simulink model "sim_quadrotor_2018"  (R2018a)
settings: Solver=ode3  StartTime=0  StopTime=inf  FixedStep=quadEDT.sampletime  MaxStep=0.1  RelTol=1e-3  EnableMultiTasking=on
InitFcn:
  | % load parameters of the default quadrotor
  | disp('Quadrotor parameters loaded by InitFcn')
  | parameters_estimationcontrol %loads mdl_quadcopter, too!
  | 
  | % change to Simulation folder if in data folder
  | %cd([matlabpath '/Simulation']);
  | cd(['C:\Users\Tony\Documents\GitHub\drone\MIT_MatlabToolbox\trunk\matlab\Simulation']);
StopFcn:
  | SimulationDataToHardwareDataFormat
values from neighbouring files (symbols this model uses):
  controlHelperParams =     [LQR_param.mat]
  dT = quadEDT.sampletime    [parameters_estimationcontrol.m]
  estimParams =     [LQR_param.mat]
  quad =     [LQR_param.mat]
  quadEDT =     [LQR_param.mat]
  sigmaW = blkdiag(0.0005, 0.1)    [parameters_estimationcontrol.m]
  sigmaX0 = zeros(2,2)    [parameters_estimationcontrol.m]
  x0 = [-0.05 0]    [parameters_estimationcontrol.m]
undefined symbols (not defined in the file or in its folder): DiscIntNeverNeededParam, Discrete, Time
libraries: simulink x28, dspswit3 x6, ctrlSharedLib x3, vrlib x1, commnoisgen2 x1
(part 1 of 2)
settings Model: Creator=Fabian Riether  LastModifiedBy=Tony
settings SolverCC: ConcurrentTasks=on  AutoInsertRateTranBlk=on
settings DataIOCC: SaveFormat=StructureWithTime  SignalLoggingSaveFormat=ModelDataLogs  SignalLogging=off  DSMLogging=off
settings OptimizationCC: ExpressionDepthLimit=2147483647  LifeSpan=1
settings DebuggingCC: UnderspecifiedInitializationDetection=Classic  MergeDetectMultiDrivingBlocksExec=none  SolverPrmCheckMsg=warning  FcnCallInpInsideContextMsg=warning  StateNameClashWarn=warning  SFUnexpectedBacktrackingDiag=warning  SFNoUnconditionalDefaultTransitionDiag=warning  SFExecutionAtInitializationDiag=none
settings HardwareCC: ProdBitPerPointer=32  ProdBitPerSizeT=32  ProdBitPerPtrDiffT=32  ProdLargestAtomicFloat=None  ProdIntDivRoundTo=Undefined  ProdEndianess=Unspecified  ProdWordSize=32  ProdHWDeviceType=32-bit Generic  TargetBitPerPointer=64  TargetBitPerSizeT=64  TargetBitPerPtrDiffT=64  TargetLongLongMode=on  TargetIntDivRoundTo=Zero  TargetEndianess=LittleEndian  TargetWordSize=64  TargetHWDeviceType=MATLAB Host  ProdEqTarget=off
settings ModelReferenceCC: PropagateSignalLabelsOutOfModel=off
settings SFSimCC: MATLABDynamicMemAlloc=off
settings RTWCC: SystemTargetFile=ert_shrlib.tlc  GenCodeOnly=on  MakeCommand="make_rtw OPTS=\"-DDEFAULT_BUFFER_SIZE=4600\""  GenerateMakefile=off  TemplateMakefile=ert_default_tmf  Description=Embedded Coder (host-based shared library target)  BuildConfiguration=Faster Runs  RTWCompilerOptimization=on
settings CodeAppCC: IgnoreCustomStorageClasses=off  StateflowObjectComments=on
settings STFCustomTargetCC: GenerateSampleERTMain=on  ParMdlRefBuildCompliant=on  CompOptLevelCompliant=on  IncludeMdlTerminateFcn=off  CombineOutputUpdateFcns=on  ERTCustomFileBanners=on  MatFileLogging=on  MultiInstanceERTCode=on  CodeInterfacePackaging=Reusable function  SupportContinuousTime=off  SupportNonInlinedSFcns=off  RemoveResetFunc=on  MATLABClassNameForMDSCustomization=Simulink.SoftwareTarget.ERTCustomization  ModelStepFunctionPrototypeControlCompliant=on  GRTInterface=off  UseToolchainInfoCompliant=on  SystemTargetFile=ert_shrlib.tlc
settings ERTTargetCC: MultiwordLength=2048  GenerateSampleERTMain=on  ConcurrentExecutionCompliant=off  IncludeMdlTerminateFcn=off  MatFileLogging=on  MultiInstanceERTCode=on  CodeInterfacePackaging=Reusable function  CPPClassGenCompliant=off  MultiInstanceErrorCode=Warning  ERTCustomFileTemplate=example_file_process.tlc  ConvertIfToSwitch=off  SuppressUnreachableDefaultCases=off
settings ConfigComp: CovMetricSettings=dw  CovHtmlReporting=on  CovSaveCumulativeToWorkspaceVar=on  CovSaveSingleToWorkspaceVar=on  CovExternalEMLEnable=off  CovSFcnEnable=off

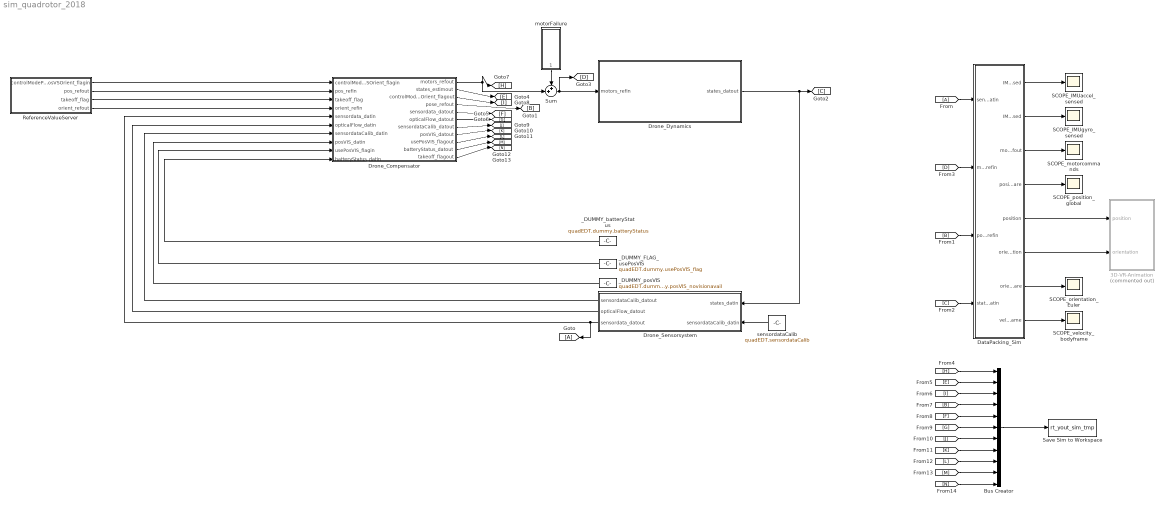
== system sim_quadrotor_2018 ==
  3D-VR-Animation : Subsystem  Commented=on
  Bus Creator : BusCreator  Inputs=11
  DataPacking_Sim : Subsystem
  Drone_Compensator : Subsystem  TreatAsAtomicUnit=on
  Drone_Dynamics : Subsystem  AncestorBlock=roblocks/Dynamics/Quadrotor
  Drone_Sensorsystem : Subsystem
  ReferenceValueServer : Subsystem
  SCOPE_IMUaccel_sensed : Scope
  SCOPE_IMUgyro_sensed : Scope
  SCOPE_motorcommands : Scope
  SCOPE_orientation_Euler : Scope
  SCOPE_position_global : Scope
  SCOPE_velocity_bodyframe : Scope
  Save Sim to Workspace : ToWorkspace  VariableName=rt_yout_sim_tmp  SaveFormat=Timeseries  SampleTime=-1
  Sum : Sum  Inputs=++|
  _DUMMY_FLAG_usePosVIS : Constant  Value=quadEDT.dummy.usePosVIS_flag
  _DUMMY_batteryStatus : Constant  Value=quadEDT.dummy.batteryStatus
  _DUMMY_posVIS : Constant  Value=quadEDT.dummy.posVIS_novisionavail
  motorFailure : Subsystem
  sensordataCalib : Constant  Value=quadEDT.sensordataCalib  SampleTime=quadEDT.sampletime
  wires:
  ReferenceValueServer/2("pos_refout ") -> Drone_Compensator/2(pos_refin)
  Sum/1 -> [D], Drone_Dynamics/1(motors_refin)
  motorFailure/1(motors_datout) -> Sum/1
  Drone_Compensator/1(motors_refout) -> [H], Sum/2
  ReferenceValueServer/1(controlModePosVSOrient_flagin) -> Drone_Compensator/1(controlModePosVSOrient_flagin)
  ReferenceValueServer/4(orient_refout) -> Drone_Compensator/4(orient_refin)
  Drone_Dynamics/1(states_datout) -> [C], Drone_Sensorsystem/1(states_datin)
  sensordataCalib/1 -> Drone_Sensorsystem/2(sensordataCalib_datin)
  Drone_Sensorsystem/2(opticalFlow_datout) -> Drone_Compensator/6(opticalFlow_datin)
  Drone_Sensorsystem/1(sensordataCalib_datout) -> Drone_Compensator/7(sensordataCalib_datin)
  Drone_Sensorsystem/3(sensordata_datout) -> [A], Drone_Compensator/5(sensordata_datin)
  _DUMMY_posVIS/1 -> Drone_Compensator/8(posVIS_datin)
  _DUMMY_FLAG_usePosVIS/1 -> Drone_Compensator/9(usePosVIS_flagin)
  _DUMMY_batteryStatus/1 -> Drone_Compensator/10(batteryStatus_datin)
  ReferenceValueServer/3("takeoff_flag ") -> Drone_Compensator/3(takeoff_flag)
  Drone_Compensator/4(pose_refout) -> [B]
  [A] -> DataPacking_Sim/1(sensordata_datin)
  [B] -> DataPacking_Sim/3(pose_refin)
  [C] -> DataPacking_Sim/4(states_datin)
  DataPacking_Sim/1(IMUaccel_sensed) -> SCOPE_IMUaccel_sensed/1
  DataPacking_Sim/2(IMUgyro_sensed) -> SCOPE_IMUgyro_sensed/1
  DataPacking_Sim/4(position_compare) -> SCOPE_position_global/1
  DataPacking_Sim/5(position) -> 3D-VR-Animation/1(position)
  DataPacking_Sim/7(orientation_compare) -> SCOPE_orientation_Euler/1
  DataPacking_Sim/6(orientation) -> 3D-VR-Animation/2(orientation)
  [D] -> DataPacking_Sim/2(motors_refin)
  DataPacking_Sim/3(motors_refout) -> SCOPE_motorcommands/1
  DataPacking_Sim/8(velocity_bodyframe) -> SCOPE_velocity_bodyframe/1
  Drone_Compensator/2(states_estimout) -> [E]
  Drone_Compensator/5(sensordata_datout) -> [F]
  Drone_Compensator/6(opticalFlow_datout) -> [G]
  Drone_Compensator/7(sensordataCalib_datout) -> [J]
  Drone_Compensator/8(posVIS_datout) -> [K]
  Drone_Compensator/9(usePosVIS_flagout) -> [L]
  Drone_Compensator/10(batteryStatus_datout) -> [M]
  [H] -> Bus Creator/1
  [E] -> Bus Creator/2
  [I] -> Bus Creator/3
  [B] -> Bus Creator/4
  [F] -> Bus Creator/5
  [G] -> Bus Creator/6
  [J] -> Bus Creator/7
  [K] -> Bus Creator/8
  [L] -> Bus Creator/9
  [M] -> Bus Creator/10
  [N] -> Bus Creator/11
  Bus Creator/1 -> Save Sim to Workspace/1
  Drone_Compensator/3(controlModePosVSOrient_flagout) -> [I]
  Drone_Compensator/11(takeoff_flagout) -> [N]

== system sim_quadrotor_2018/3D-VR-Animation ==
  note: Student contribution by Erlend Solbakk Harbitz
  note: In animation:
      | X-axis: red
      | Y-axis: green
      | Z-axis: blue
  note: Animation
  note: Positions = [X; Y; Z] (Inertia frame with Z-axis downwards)
      | Theta      = [yaw (psi); pitch ( theta); roll (phi) ]
      |
      | Euler angles scheme: First yaw, then pitch, then roll
  position : Inport
  orientation : Inport  Port=2
  Double click for animation : vrlib/VR Sink  RequirementInfo={} %GIDa_850cb678_ba1c_4e80_94b9_fad132a707ef  InstantiateOnLoad=on  SampleTime=0.1  ViewEnable=on  RemoteChange=off  RemoteView=off  FieldsWritten=DRONE.translation.3.1.1.double#roll_rotation.rotation.4.1.1.double#pitch_rotation.rotation.4.1.1.double#yaw_rotation.rotation.4.1.1.double  WorldFileName=Animation/DroneWorld.wrl  AutoView=off  VideoDimensions=[]  AllowVariableSize=off
      settings: SourceProductBaseCode=VR
  Euler angle rotations : MATLAB Function  TreatAsAtomicUnit=on
  Rate Transition : RateTransition
  Rate Transition1 : RateTransition
  wires:
  orientation/1 -> Rate Transition1/1  "Euler angles (yaw, pitch, roll)"
  position/1 -> Rate Transition/1  "Inertia positions X,Y,Z"
  Rate Transition1/1 -> Euler angle rotations/1(O)
  Rate Transition/1 -> Double click for animation/1
  Euler angle rotations/1(rot_phi) -> Double click for animation/2  "Third rotation"
  Euler angle rotations/2(rot_theta) -> Double click for animation/3  "Second rotation"
  Euler angle rotations/3(rot_psi) -> Double click for animation/4  "First rotation"

== system sim_quadrotor_2018/DataPacking_Sim ==
  sensordata_datin : Inport
  motors_refin : Inport  Port=2
  pose_refin : Inport  Port=3
  states_datin : Inport  Port=4
  Augment/Mux Signals : Subsystem
  Bus Selector1 : BusSelector  OutputSignals=dx,dy,dz  OutputAsBus=on
  Bus Selector6 : BusSelector  OutputSignals=ddx,ddy,ddz  OutputAsBus=on
  Bus Selector9 : BusSelector  OutputSignals=p,q,r  OutputAsBus=on
  IMUaccel_sensed : Outport
  IMUgyro_sensed : Outport  Port=2
  motors_refout : Outport  Port=3
  position_compare : Outport  Port=4
  position : Outport  Port=5
  orientation : Outport  Port=6
  orientation_compare : Outport  Port=7
  velocity_bodyframe : Outport  Port=8
  wires:
  sensordata_datin/1 -> Bus Selector6/1, Bus Selector9/1
  states_datin/1 -> Bus Selector1/1, Augment/Mux Signals/2(states_datin)
  pose_refin/1 -> Augment/Mux Signals/1(pose_refin)
  Bus Selector9/1 -> IMUgyro_sensed/1
  Bus Selector6/1 -> IMUaccel_sensed/1
  Augment/Mux Signals/1(position_compare_datout) -> position_compare/1
  Augment/Mux Signals/2(position_datout) -> position/1
  Augment/Mux Signals/3(orientation_compare_datout) -> orientation_compare/1
  Augment/Mux Signals/4(orientation_datout) -> orientation/1
  motors_refin/1 -> motors_refout/1
  Bus Selector1/1 -> velocity_bodyframe/1

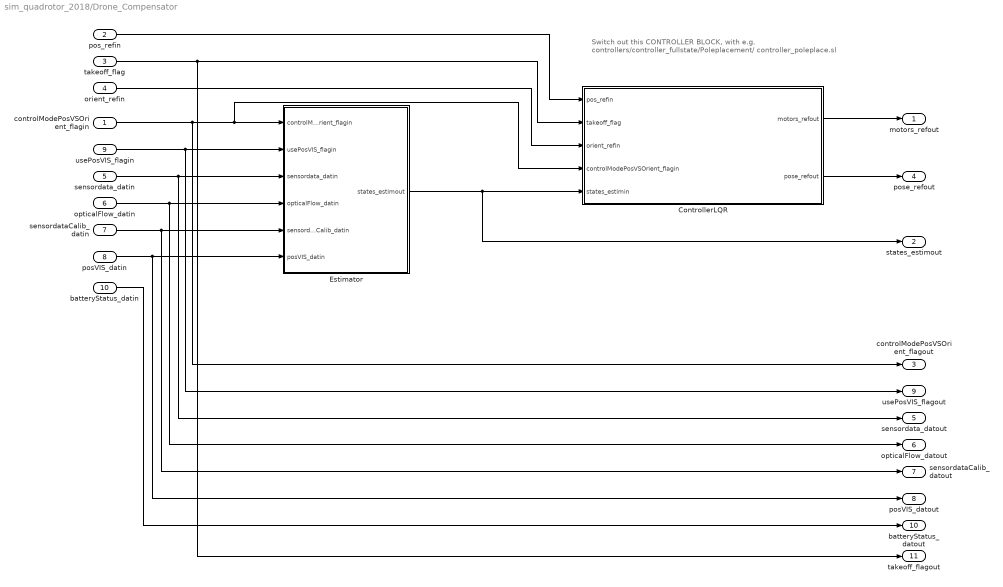
== system sim_quadrotor_2018/Drone_Compensator ==
  note: Switch out this CONTROLLER BLOCK, with e.g.
      | controllers/controller_fullstate/Poleplacement/
      | controller_poleplace.sl
  controlModePosVSOrient_flagin : Inport
  pos_refin : Inport  Port=2
  takeoff_flag : Inport  Port=3
  orient_refin : Inport  Port=4
  sensordata_datin : Inport  Port=5
  opticalFlow_datin : Inport  Port=6
  sensordataCalib_datin : Inport  Port=7
  posVIS_datin : Inport  Port=8
  usePosVIS_flagin : Inport  Port=9
  batteryStatus_datin : Inport  Port=10
  ControllerLQR : Subsystem  TreatAsAtomicUnit=on
  Estimator : Subsystem
  motors_refout : Outport
  states_estimout : Outport  Port=2
  controlModePosVSOrient_flagout : Outport  Port=3
  pose_refout : Outport  Port=4
  sensordata_datout : Outport  Port=5
  opticalFlow_datout : Outport  Port=6
  sensordataCalib_datout : Outport  Port=7
  posVIS_datout : Outport  Port=8
  usePosVIS_flagout : Outport  Port=9
  batteryStatus_datout : Outport  Port=10
  takeoff_flagout : Outport  Port=11
  wires:
  sensordata_datin/1 -> sensordata_datout/1, Estimator/3(sensordata_datin)
  pos_refin/1 -> ControllerLQR/1(pos_refin)
  Estimator/1(states_estimout) -> ControllerLQR/5(states_estimin), states_estimout/1
  orient_refin/1 -> ControllerLQR/3(orient_refin)
  controlModePosVSOrient_flagin/1 -> controlModePosVSOrient_flagout/1, ControllerLQR/4(controlModePosVSOrient_flagin), Estimator/1(controlModePosVSOrient_flagin)
  sensordataCalib_datin/1 -> sensordataCalib_datout/1, Estimator/5(sensordataCalib_datin)
  opticalFlow_datin/1 -> opticalFlow_datout/1, Estimator/4(opticalFlow_datin)
  posVIS_datin/1 -> posVIS_datout/1, Estimator/6(posVIS_datin)
  ControllerLQR/1(motors_refout) -> motors_refout/1
  usePosVIS_flagin/1 -> usePosVIS_flagout/1, Estimator/2(usePosVIS_flagin)
  ControllerLQR/2(pose_refout) -> pose_refout/1
  batteryStatus_datin/1 -> batteryStatus_datout/1
  takeoff_flag/1 -> ControllerLQR/2(takeoff_flag), takeoff_flagout/1

== system sim_quadrotor_2018/Drone_Dynamics ==
  motors_refin : Inport
  Bus Creator : BusCreator  Inputs='X','Y','Z','yaw','pitch','roll','dx','dy','dz','p','q','r'
  Demux : Demux  Outputs=12
  Dynamics (Robotics Toolbox Peter Corke) : S-Function  FunctionName=quadrotor_dynamics  Parameters=quad  SFunctionDeploymentMode=off  EnableBusSupport=off
  MotorsToW : Subsystem
  Rate Transition : RateTransition
  states_datout : Outport
  wires:
  Demux/1 -> Bus Creator/1  "X"
  Demux/3 -> Bus Creator/3  "Z"
  Demux/4 -> Bus Creator/4  "yaw"
  Demux/5 -> Bus Creator/5  "pitch"
  motors_refin/1 -> Rate Transition/1
  Demux/7 -> Bus Creator/7  "dx"
  Demux/9 -> Bus Creator/9  "dz"
  Demux/2 -> Bus Creator/2  "Y"
  Demux/6 -> Bus Creator/6  "roll"
  Demux/8 -> Bus Creator/8  "dy"
  Bus Creator/1 -> states_datout/1
  Dynamics (Robotics Toolbox Peter Corke)/1 -> Demux/1
  Demux/10 -> Bus Creator/10  "p"
  Demux/11 -> Bus Creator/11  "q"
  Demux/12 -> Bus Creator/12  "r"
  MotorsToW/1(omegas_datout) -> Dynamics (Robotics Toolbox Peter Corke)/1
  Rate Transition/1 -> MotorsToW/1(motors_datin)

== system sim_quadrotor_2018/Drone_Sensorsystem ==
  states_datin : Inport
  sensordataCalib_datin : Inport  Port=2
  IMU_Pressure : Subsystem
  Rate Transition1 : RateTransition  OutPortSampleTime=quadEDT.sampletime
  Rate Transition2 : RateTransition  OutPortSampleTime=quadEDT.sampletime
  camera : Subsystem
  sensordataCalib_datout : Outport
  opticalFlow_datout : Outport  Port=2
  sensordata_datout : Outport  Port=3
  wires:
  states_datin/1 -> IMU_Pressure/2(states_datin), camera/1(states_datin)
  sensordataCalib_datin/1 -> sensordataCalib_datout/1, IMU_Pressure/1(sensordataCalib_datin)
  Rate Transition2/1 -> sensordata_datout/1
  Rate Transition1/1 -> opticalFlow_datout/1
  IMU_Pressure/1(sensordata_datout) -> Rate Transition2/1
  camera/1(opticalFlow_datout) -> Rate Transition1/1

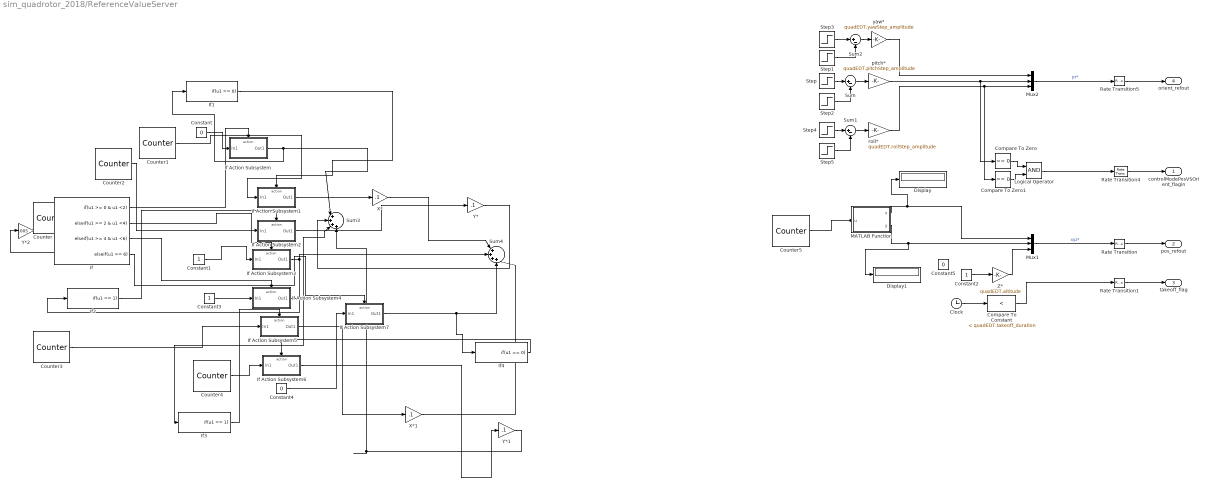
== system sim_quadrotor_2018/ReferenceValueServer ==
  Clock : Clock
  Compare To Constant : simulink/Logic and Bit Operations/Compare To Constant  relop=<  const=quadEDT.takeoff_duration  OutDataTypeStr=boolean
  Compare To Zero : simulink/Logic and Bit Operations/Compare To Zero  relop===  OutDataTypeStr=boolean
  Compare To Zero1 : simulink/Logic and Bit Operations/Compare To Zero  relop===  OutDataTypeStr=boolean
  Constant : Constant  Value=0  SampleTime=0
  Constant1 : Constant  SampleTime=0
  Constant2 : Constant  SampleTime=0
  Constant3 : Constant  SampleTime=0
  Constant4 : Constant  Value=0  SampleTime=0
  Constant5 : Constant  Value=0  SampleTime=0
  Counter : dspswit3/Counter  Direction=Up  CountEvent=Free running  CounterSize=User defined  MaxCount=1600  InitialCount=0  Output=Count  HitValue=32  ResetInput=on  SamplesPerFrame=1  Ts=.005  CntDtype=double  HitDtype=Logical
  Counter1 : dspswit3/Counter  Direction=Up  CountEvent=Free running  CounterSize=User defined  MaxCount=10  InitialCount=0  Output=Count  HitValue=32  ResetInput=on  SamplesPerFrame=1  Ts=.005  CntDtype=double  HitDtype=Logical
  Counter2 : dspswit3/Counter  Direction=Up  CountEvent=Free running  CounterSize=User defined  MaxCount=10  InitialCount=0  Output=Count  HitValue=32  ResetInput=on  SamplesPerFrame=1  Ts=.005  CntDtype=double  HitDtype=Logical
  Counter3 : dspswit3/Counter  Direction=Down  CountEvent=Free running  CounterSize=User defined  MaxCount=10  InitialCount=10  Output=Count  HitValue=32  ResetInput=on  SamplesPerFrame=1  Ts=.005  CntDtype=double  HitDtype=Logical
  Counter4 : dspswit3/Counter  Direction=Down  CountEvent=Free running  CounterSize=User defined  MaxCount=10  InitialCount=10  Output=Count  HitValue=32  ResetInput=on  SamplesPerFrame=1  Ts=.005  CntDtype=double  HitDtype=Logical
  Counter5 : dspswit3/Counter  Direction=Up  CountEvent=Free running  CounterSize=User defined  MaxCount=10000000000000000000000000000000000000000  InitialCount=0  Output=Count  HitValue=32  ResetInput=off  SamplesPerFrame=1  Ts=.005  CntDtype=double  HitDtype=Logical
  Display : Display
      settings: Decimation=2
  Display1 : Display
      settings: Decimation=2
  If : If  IfExpression=u1 >= 0 & u1 <2  ElseIfExpressions=u1 >= 2 & u1 <4,u1 >= 4 & u1 <6,u1 >= 6  ShowElse=off
  If Action Subsystem : Subsystem  TreatAsAtomicUnit=on
  If Action Subsystem1 : Subsystem  TreatAsAtomicUnit=on
  If Action Subsystem2 : Subsystem  TreatAsAtomicUnit=on
  If Action Subsystem3 : Subsystem  TreatAsAtomicUnit=on
  If Action Subsystem4 : Subsystem  TreatAsAtomicUnit=on
  If Action Subsystem5 : Subsystem  TreatAsAtomicUnit=on
  If Action Subsystem6 : Subsystem  TreatAsAtomicUnit=on
  If Action Subsystem7 : Subsystem  TreatAsAtomicUnit=on
  If1 : If  IfExpression=u1 == 0  ShowElse=off
  If2 : If  IfExpression=u1 == 1  ShowElse=off
  If3 : If  IfExpression=u1 == 1  ShowElse=off
  If4 : If  IfExpression=u1 == 0  ShowElse=off
  Logical Operator : Logic  AllPortsSameDT=off  OutDataTypeStr=boolean
  MATLAB Function : MATLAB Function  TreatAsAtomicUnit=on
  Mux1 : Mux  Inputs=3
  Mux2 : Mux  Inputs=3
  Rate Transition{,1,4..5} (4 alike) : RateTransition  OutPortSampleTime=quadEDT.sampletime
  Step : Step  Time=quadEDT.pitchStep_time  SampleTime=0
  Step1 : Step  Time=quadEDT.yawStep_time+quadEDT.yawStep_duration  SampleTime=0
  Step2 : Step  Time=quadEDT.pitchStep_time+quadEDT.pitchStep_duration  SampleTime=0
  Step3 : Step  Time=quadEDT.yawStep_time  SampleTime=0
  Step4 : Step  Time=quadEDT.rollStep_time  SampleTime=0
  Step5 : Step  Time=quadEDT.rollStep_duration+quadEDT.rollStep_time  SampleTime=0
  Sum : Sum  Inputs=|+-
  Sum1 : Sum  Inputs=|+-
  Sum2 : Sum  Inputs=|+-
  Sum3 : Sum  Inputs=|++++
  Sum4 : Sum  Inputs=|++++
  X* : Gain  Gain=.1
  X*1 : Gain  Gain=.1
  Y* : Gain  Gain=.1
  Y*1 : Gain  Gain=.1
  Y*2 : Gain  Gain=.005
  Z* : Gain  Gain=quadEDT.altitude
  pitch* : Gain  Gain=quadEDT.pitchStep_amplitude
  roll* : Gain  Gain=quadEDT.rollStep_amplitude
  yaw* : Gain  Gain=quadEDT.yawStep_amplitude
  controlModePosVSOrient_flagin : Outport
  "pos_refout " : Outport  Port=2
  "takeoff_flag " : Outport  Port=3
  orient_refout : Outport  Port=4
  wires:
  Constant/1 -> If Action Subsystem/1(In1)
  Mux1/1 -> Rate Transition/1  "xyz*"
  Rate Transition/1 -> "pos_refout "/1
  Rate Transition4/1 -> controlModePosVSOrient_flagin/1
  Step/1 -> Sum/1
  Mux2/1 -> Rate Transition5/1  "pr*"
  Sum1/1 -> roll*/1
  Rate Transition5/1 -> orient_refout/1
  Sum/1 -> pitch*/1
  Step2/1 -> Sum/2
  yaw*/1 -> Mux2/1
  pitch*/1 -> Mux2/2, Compare To Zero/1
  roll*/1 -> Mux2/3, Compare To Zero1/1
  Compare To Zero/1 -> Logical Operator/1
  Compare To Zero1/1 -> Logical Operator/2
  Logical Operator/1 -> Rate Transition4/1
  Clock/1 -> Compare To Constant/1
  Constant2/1 -> Z*/1
  Z*/1 -> Mux1/3
  Step4/1 -> Sum1/1
  Step5/1 -> Sum1/2
  Sum2/1 -> yaw*/1
  Step3/1 -> Sum2/1
  Step1/1 -> Sum2/2
  Compare To Constant/1 -> Rate Transition1/1
  Rate Transition1/1 -> "takeoff_flag "/1
  Constant1/1 -> If Action Subsystem3/1(In1)
  If Action Subsystem/1(Out1) -> If1/1, Sum3/1
  If Action Subsystem1/1(Out1) -> X*/1
  Counter/1 -> Y*2/1
  Counter1/1 -> If Action Subsystem1/1(In1)
  If/1 -> If Action Subsystem/Action
  Counter2/1 -> If Action Subsystem2/1(In1)
  If/2 -> If Action Subsystem3/Action
  If Action Subsystem3/1(Out1) -> If2/1, Sum4/2
  If Action Subsystem2/1(Out1) -> Y*/1
  If/3 -> If Action Subsystem4/Action
  Constant3/1 -> If Action Subsystem4/1(In1)
  Counter3/1 -> If Action Subsystem5/1(In1)
  If Action Subsystem4/1(Out1) -> If3/1, Sum3/3
  If Action Subsystem5/1(Out1) -> X*1/1
  If/4 -> If Action Subsystem7/Action
  Counter4/1 -> If Action Subsystem6/1(In1)
  If Action Subsystem6/1(Out1) -> Y*1/1
  If Action Subsystem7/1(Out1) -> If4/1, Sum4/4
  Constant4/1 -> If Action Subsystem7/1(In1)
  If1/1 -> If Action Subsystem1/Action
  If2/1 -> If Action Subsystem2/Action
  If3/1 -> If Action Subsystem5/Action
  If4/1 -> If Action Subsystem6/Action
  X*/1 -> Sum4/1
  X*1/1 -> Sum4/3
  Y*/1 -> Sum3/2
  Y*1/1 -> Sum3/4
  Y*2/1 -> If/1
  Counter5/1 -> MATLAB Function/1(u)
  MATLAB Function/2(y) -> Display1/1, Mux1/2
  MATLAB Function/1(x) -> Display/1, Mux1/1

== system sim_quadrotor_2018/motorFailure ==
  Mux1 : Mux
  Step : Step  Time=quadEDT.motorFailure_time  SampleTime=quadEDT.sampletime
  Step1 : Step  Time=quadEDT.motorFailure_time + quadEDT.motorFailure_duration  SampleTime=quadEDT.sampletime
  Sum : Sum  Inputs=|+-
  motorFailure_gainm1 : Gain  Gain=quadEDT.motorFailure_m2
  motorFailure_gainm2 : Gain  Gain=quadEDT.motorFailure_m2
  motorFailure_gainm3 : Gain  Gain=quadEDT.motorFailure_m3
  motorFailure_gainm4 : Gain  Gain=quadEDT.motorFailure_m3
  motors_datout : Outport
  wires:
  Step/1 -> Sum/1
  Step1/1 -> Sum/2
  Sum/1 -> motorFailure_gainm1/1, motorFailure_gainm2/1, motorFailure_gainm3/1, motorFailure_gainm4/1
  motorFailure_gainm2/1 -> Mux1/2
  motorFailure_gainm3/1 -> Mux1/3
  motorFailure_gainm4/1 -> Mux1/4
  motorFailure_gainm1/1 -> Mux1/1
  Mux1/1 -> motors_datout/1

== system sim_quadrotor_2018/DataPacking_Sim/Augment//Mux Signals ==
  pose_refin : Inport
  states_datin : Inport  Port=2
  Bus Selector7 : BusSelector  OutputSignals=X,Y,Z  OutputAsBus=on
  Bus Selector8 : BusSelector  OutputSignals=yaw,pitch,roll  OutputAsBus=on
  Mux : Mux  Inputs=2
  Mux1 : Mux  Inputs=2
  Rate Transition : RateTransition
  orientation_ref : Selector  InputPortWidth=6  IndexOptions=Index vector (dialog)  Indices=[4:6]  OutputSizes=1
  position_ref : Selector  InputPortWidth=6  IndexOptions=Index vector (dialog)  Indices=[1:3]  OutputSizes=1
  position_compare_datout : Outport
  position_datout : Outport  Port=2
  orientation_compare_datout : Outport  Port=3
  orientation_datout : Outport  Port=4
  wires:
  states_datin/1 -> Bus Selector7/1, Bus Selector8/1
  Rate Transition/1 -> orientation_ref/1, position_ref/1
  pose_refin/1 -> Rate Transition/1
  Bus Selector8/1 -> orientation_datout/1, Mux1/2
  Mux1/1 -> orientation_compare_datout/1
  position_ref/1 -> Mux/1
  Mux/1 -> position_compare_datout/1
  orientation_ref/1 -> Mux1/1
  Bus Selector7/1 -> position_datout/1, Mux/2

== system sim_quadrotor_2018/Drone_Compensator/ControllerLQR ==
  pos_refin : Inport
  takeoff_flag : Inport  Port=2
  orient_refin : Inport  Port=3
  controlModePosVSOrient_flagin : Inport  Port=4
  states_estimin : Inport  Port=5
  Add : Sum  Inputs=-+
  FullstateController : Subsystem
  Select pose : Selector  InputPortWidth=12  IndexOptions=Index vector (dialog)  Indices=[1:6]  OutputSizes=1
  SysteminputConverter : Subsystem
  statesReferences : Subsystem
  motors_refout : Outport
  pose_refout : Outport  Port=2
  wires:
  Select pose/1 -> pose_refout/1
  statesReferences/1(states_refout) -> Add/1, Select pose/1
  controlModePosVSOrient_flagin/1 -> statesReferences/3(controlModePosVSOrient_flagin)
  states_estimin/1 -> statesReferences/4(states_estimin), Add/2
  orient_refin/1 -> statesReferences/2(orient_refin)
  pos_refin/1 -> statesReferences/1(pos_refin)
  Add/1 -> FullstateController/1(state_error_datin)  "state error e"
  FullstateController/1(motors_refout) -> SysteminputConverter/2(motors_refin)
  SysteminputConverter/1(motors_refout) -> motors_refout/1
  takeoff_flag/1 -> SysteminputConverter/1(takeoffphase_flagin)

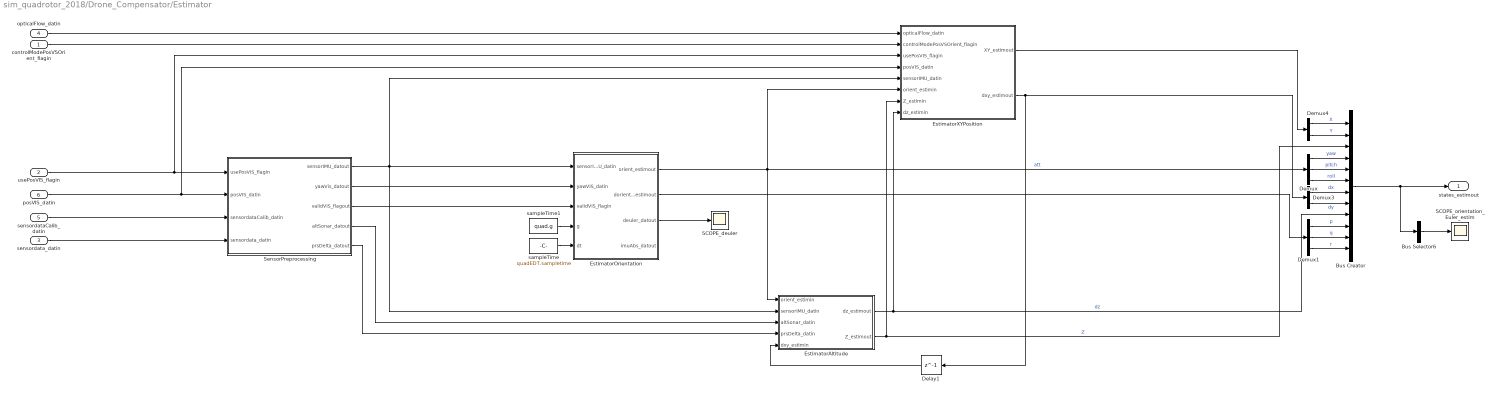
== system sim_quadrotor_2018/Drone_Compensator/Estimator ==
  controlModePosVSOrient_flagin : Inport
  usePosVIS_flagin : Inport  Port=2
  sensordata_datin : Inport  Port=3
  opticalFlow_datin : Inport  Port=4
  sensordataCalib_datin : Inport  Port=5
  posVIS_datin : Inport  Port=6
  Bus Creator : BusCreator  Inputs='X','Y','Z','yaw','pitch','roll','dx','dy','dz','p','q','r'
  Bus Selector6 : BusSelector  OutputSignals=yaw,pitch,roll  OutputAsBus=on
  Delay1 : Delay  DelayLength=1  InitialCondition=0
  Demux : Demux  Outputs=3
  Demux1 : Demux  Outputs=3
  Demux3 : Demux  Outputs=2
  Demux4 : Demux  Outputs=2
  EstimatorAltitude : Subsystem
  EstimatorOrientation : MATLAB Function  TreatAsAtomicUnit=on
  EstimatorXYPosition : Subsystem
  SCOPE_deuler : Scope
  SCOPE_orientation_Euler_estim : Scope
  SensorPreprocessing : Subsystem
  sampleTime : Constant  Value=quadEDT.sampletime  SampleTime=quadEDT.sampletime
  sampleTime1 : Constant  Value=quad.g  SampleTime=quadEDT.sampletime
  states_estimout : Outport
  wires:
  Bus Creator/1 -> Bus Selector6/1, states_estimout/1
  sampleTime/1 -> EstimatorOrientation/5(dt)
  sensordataCalib_datin/1 -> SensorPreprocessing/3(sensordataCalib_datin)
  EstimatorAltitude/2(Z_estimout) -> Bus Creator/3, EstimatorXYPosition/7(Z_estimin)  "Z"
  EstimatorAltitude/1(dz_estimout) -> EstimatorXYPosition/8(dz_estimin), Bus Creator/9  "dz"
  opticalFlow_datin/1 -> EstimatorXYPosition/1(opticalFlow_datin)
  Demux3/1 -> Bus Creator/7  "dx"
  Demux3/2 -> Bus Creator/8  "dy"
  EstimatorXYPosition/2(dxy_estimout) -> Delay1/1, Demux3/1
  Delay1/1 -> EstimatorAltitude/5(dxy_estimin)
  controlModePosVSOrient_flagin/1 -> EstimatorXYPosition/2(controlModePosVSOrient_flagin)
  Demux4/1 -> Bus Creator/1  "X"
  Demux4/2 -> Bus Creator/2  "Y"
  EstimatorXYPosition/1(XY_estimout) -> Demux4/1
  posVIS_datin/1 -> EstimatorXYPosition/4(posVIS_datin), SensorPreprocessing/2(posVIS_datin)
  usePosVIS_flagin/1 -> SensorPreprocessing/1(usePosVIS_flagin), EstimatorXYPosition/3(usePosVIS_flagin)
  Bus Selector6/1 -> SCOPE_orientation_Euler_estim/1
  SensorPreprocessing/1(sensorIMU_datout) -> EstimatorAltitude/2(sensorIMU_datin), EstimatorOrientation/1(sensorIMU_datin), EstimatorXYPosition/5(sensorIMU_datin)
  sensordata_datin/1 -> SensorPreprocessing/4(sensordata_datin)
  SensorPreprocessing/4(altSonar_datout) -> EstimatorAltitude/3(altSonar_datin)
  SensorPreprocessing/5(prsDelta_datout) -> EstimatorAltitude/4(prsDelta_datin)
  EstimatorOrientation/1(orient_estimout) -> EstimatorAltitude/1(orient_estimin), EstimatorXYPosition/6(orient_estimin), Demux/1  "att"
  Demux/2 -> Bus Creator/5  "pitch"
  Demux1/1 -> Bus Creator/10  "p"
  Demux1/2 -> Bus Creator/11  "q"
  Demux1/3 -> Bus Creator/12  "r"
  EstimatorOrientation/2(dorient_estimout) -> Demux1/1
  SensorPreprocessing/3(validVIS_flagout) -> EstimatorOrientation/3(validVIS_flagin)
  SensorPreprocessing/2(yawVis_datout) -> EstimatorOrientation/2(yawVIS_datin)
  Demux/3 -> Bus Creator/6  "roll"
  Demux/1 -> Bus Creator/4  "yaw"
  EstimatorOrientation/3(deuler_datout) -> SCOPE_deuler/1
  sampleTime1/1 -> EstimatorOrientation/4(g)

== system sim_quadrotor_2018/Drone_Dynamics/MotorsToW ==
  motors_datin : Inport
  Gain : Gain  Gain=quadEDT.motorUnknownGain_gain
  Motordirections : Gain  Gain=[1 -1 1 -1]
  Motordirections1 : Gain  Gain=[1 -1 1 -1]
  Saturation5 : Saturate  UpperLimit=quadEDT.motors_max  LowerLimit=10
  Signed Sqrt : Sqrt  Operator=signedSqrt  SaturateOnIntegerOverflow=on
  motorsToW2_Gain : Gain  Gain=quadEDT.motorcommandToW2_gain
  omegas_datout : Outport
  wires:
  motorsToW2_Gain/1 -> Signed Sqrt/1
  Signed Sqrt/1 -> Gain/1
  motors_datin/1 -> Motordirections/1
  Motordirections/1 -> Saturation5/1
  Saturation5/1 -> Motordirections1/1
  Motordirections1/1 -> motorsToW2_Gain/1
  Gain/1 -> omegas_datout/1

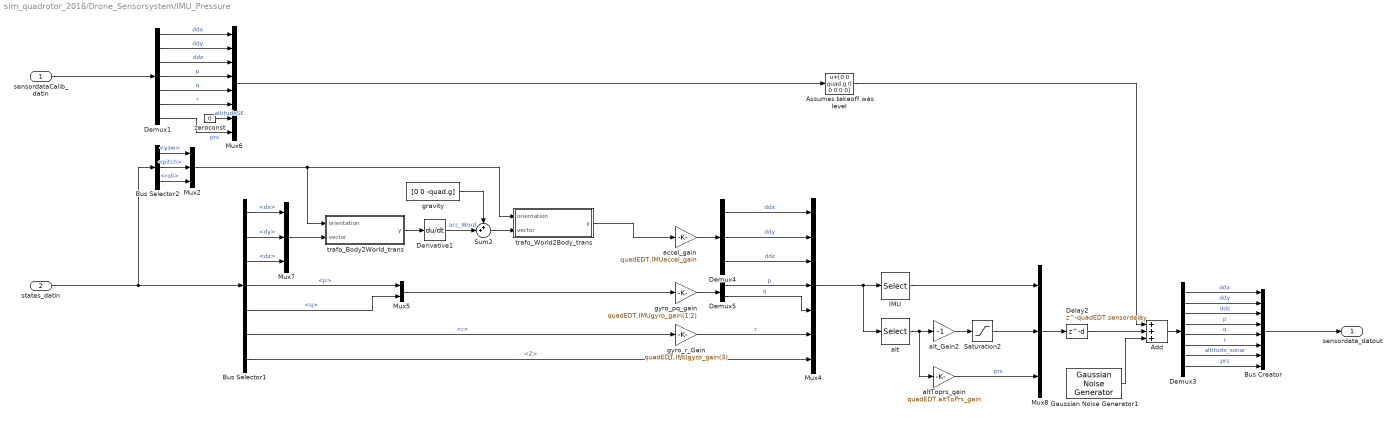
== system sim_quadrotor_2018/Drone_Sensorsystem/IMU_Pressure ==
  sensordataCalib_datin : Inport
  states_datin : Inport  Port=2
  Add : Sum  Inputs=+++
  Assumes takeoff was level : Bias  Bias=[0 0 quad.g 0 0 0 0 0]
  Bus Creator : BusCreator  Inputs=8
  Bus Selector1 : BusSelector  OutputSignals=dx,dy,dz,p,q,r,Z
  Bus Selector2 : BusSelector  OutputSignals=yaw,pitch,roll
  Delay2 : Delay  DelayLength=quadEDT.sensordelay  InitialCondition=0
  Demux1 : Demux  Outputs=7
  Demux3 : Demux  Outputs=8
  Demux4 : Demux  Outputs=3
  Demux5 : Demux  Outputs=2
  Derivative1 : Derivative
  Gaussian Noise Generator1 : commnoisgen2/Gaussian Noise Generator  m=0  d=quadEDT.noiseSensed_var  s=41  Ts=quadEDT.sampletime  frameBased=off  sampPerFrame=1  orient=off  outDataType=double
  IMU : Selector  InputPortWidth=7  IndexOptions=Index vector (dialog)  Indices=[1:6]  OutputSizes=1
  Mux2 : Mux  Inputs=3
  Mux4 : Mux  Inputs=7
  Mux5 : Mux  Inputs=2
  Mux6 : Mux  Inputs=8
  Mux7 : Mux  Inputs=3
  Mux8 : Mux  Inputs=3
  Saturation2 : Saturate  UpperLimit=inf  LowerLimit=quadEDT.altSenor_min
  Sum2 : Sum  Inputs=++|
  accel_gain : Gain  Gain=quadEDT.IMUaccel_gain
  alt : Selector  InputPortWidth=7  IndexOptions=Index vector (dialog)  Indices=[7]  OutputSizes=1
  altToprs_gain : Gain  Gain=quadEDT.altToPrs_gain
  alt_Gain2 : Gain  Gain=-1
  gravity : Constant  Value=[0 0 -quad.g]
  gyro_pq_gain : Gain  Gain=quadEDT.IMUgyro_gain(1:2)
  gyro_r_Gain : Gain  Gain=quadEDT.IMUgyro_gain(3)
  trafo_Body2World_trans : MATLAB Function  TreatAsAtomicUnit=on
  trafo_World2Body_trans : MATLAB Function  TreatAsAtomicUnit=on
  zeroconst : Constant  Value=0
  sensordata_datout : Outport
  wires:
  sensordataCalib_datin/1 -> Demux1/1
  Bus Selector2/1 -> Mux2/1  "<yaw>"
  Bus Selector2/2 -> Mux2/2  "<pitch>"
  Bus Selector2/3 -> Mux2/3  "<roll>"
  Demux1/1 -> Mux6/1  "ddx"
  Demux1/2 -> Mux6/2  "ddy"
  Demux1/3 -> Mux6/3  "ddz"
  Demux1/4 -> Mux6/4  "p"
  Demux1/5 -> Mux6/5  "q"
  Demux1/6 -> Mux6/6  "r"
  zeroconst/1 -> Mux6/7  "altitudeSE"
  Demux1/7 -> Mux6/8  "prs"
  Mux6/1 -> Assumes takeoff was level/1
  Add/1 -> Demux3/1
  Demux3/3 -> Bus Creator/3  "ddz"
  Demux3/1 -> Bus Creator/1  "ddx"
  Demux3/2 -> Bus Creator/2  "ddy"
  Demux3/4 -> Bus Creator/4  "p"
  Demux3/5 -> Bus Creator/5  "q"
  Demux3/6 -> Bus Creator/6  "r"
  Demux3/7 -> Bus Creator/7  "altitude_sonar"
  Demux3/8 -> Bus Creator/8  "prs"
  Bus Creator/1 -> sensordata_datout/1
  Delay2/1 -> Add/2
  Assumes takeoff was level/1 -> Add/1
  Demux5/2 -> Mux4/5  "q"
  Demux5/1 -> Mux4/4  "p"
  states_datin/1 -> Bus Selector1/1, Bus Selector2/1
  Bus Selector1/2 -> Mux7/2  "<dy>"
  trafo_World2Body_trans/1(y) -> accel_gain/1
  Demux4/1 -> Mux4/1  "ddx"
  Demux4/2 -> Mux4/2  "ddy"
  gyro_r_Gain/1 -> Mux4/6  "r"
  Demux4/3 -> Mux4/3  "ddz"
  gravity/1 -> Sum2/1
  Bus Selector1/4 -> Mux5/1  "<p>"
  Bus Selector1/5 -> Mux5/2  "<q>"
  Bus Selector1/6 -> gyro_r_Gain/1  "<r>"
  Bus Selector1/7 -> Mux4/7  "<Z>"
  Bus Selector1/3 -> Mux7/3  "<dz>"
  Mux5/1 -> gyro_pq_gain/1
  Bus Selector1/1 -> Mux7/1  "<dx>"
  accel_gain/1 -> Demux4/1
  gyro_pq_gain/1 -> Demux5/1
  Mux7/1 -> trafo_Body2World_trans/2(vector)
  trafo_Body2World_trans/1(y) -> Derivative1/1
  Sum2/1 -> trafo_World2Body_trans/2(vector)
  Derivative1/1 -> Sum2/2  "acc_Word"
  Mux4/1 -> IMU/1, alt/1
  alt/1 -> altToprs_gain/1, alt_Gain2/1
  alt_Gain2/1 -> Saturation2/1
  IMU/1 -> Mux8/1
  Saturation2/1 -> Mux8/2
  Mux8/1 -> Delay2/1
  Mux2/1 -> trafo_Body2World_trans/1(orientation), trafo_World2Body_trans/1(orientation)
  altToprs_gain/1 -> Mux8/3  "prs"
  Gaussian Noise Generator1/1 -> Add/3

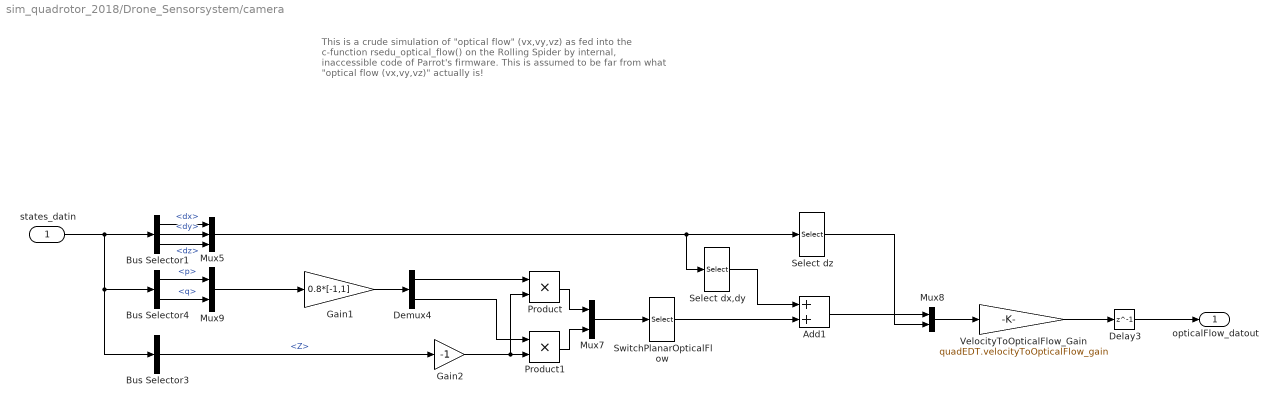
== system sim_quadrotor_2018/Drone_Sensorsystem/camera ==
  note: This is a crude simulation of "optical flow" (vx,vy,vz) as
      | fed into the c-function rsedu_optical_flow() on the Rolling Spider
      | by internal, inaccessible code of Parrot's firmware.
      | This is assumed to be far from what "optical flow (vx,vy,vz)" actually is!
  states_datin : Inport
  Add1 : Sum
  Bus Selector1 : BusSelector  OutputSignals=dx,dy,dz
  Bus Selector3 : BusSelector  OutputSignals=Z
  Bus Selector4 : BusSelector  OutputSignals=p,q
  Delay3 : Delay  DelayLength=1  InitialCondition=0
  Demux4 : Demux  Outputs=2
  Gain1 : Gain  Gain=0.8*[-1,1]
  Gain2 : Gain  Gain=-1
  Mux5 : Mux  Inputs=3
  Mux7 : Mux  Inputs=2
  Mux8 : Mux  Inputs=2
  Mux9 : Mux  Inputs=2
  Product : Product
  Product1 : Product
  Select dx,dy : Selector  InputPortWidth=3  IndexOptions=Index vector (dialog)  Indices=[1 2]  OutputSizes=1
  Select dz : Selector  InputPortWidth=3  IndexOptions=Index vector (dialog)  Indices=3  OutputSizes=1
  SwitchPlanarOpticalFlow : Selector  InputPortWidth=2  IndexOptions=Index vector (dialog)  Indices=[2 1]  OutputSizes=1
  VelocityToOpticalFlow_Gain : Gain  Gain=quadEDT.velocityToOpticalFlow_gain
  opticalFlow_datout : Outport
  wires:
  states_datin/1 -> Bus Selector3/1, Bus Selector4/1, Bus Selector1/1
  Bus Selector1/1 -> Mux5/1  "<dx>"
  Bus Selector1/2 -> Mux5/2  "<dy>"
  Bus Selector1/3 -> Mux5/3  "<dz>"
  VelocityToOpticalFlow_Gain/1 -> Delay3/1
  Mux5/1 -> Select dx,dy/1, Select dz/1
  Demux4/1 -> Product/1
  Gain1/1 -> Demux4/1
  Demux4/2 -> Product1/1
  Product/1 -> Mux7/1
  Product1/1 -> Mux7/2
  Mux7/1 -> SwitchPlanarOpticalFlow/1
  Mux9/1 -> Gain1/1
  Gain2/1 -> Product/2, Product1/2
  Select dx,dy/1 -> Add1/1
  SwitchPlanarOpticalFlow/1 -> Add1/2
  Add1/1 -> Mux8/1
  Select dz/1 -> Mux8/2
  Bus Selector3/1 -> Gain2/1  "<Z>"
  Bus Selector4/1 -> Mux9/1  "<p>"
  Bus Selector4/2 -> Mux9/2  "<q>"
  Mux8/1 -> VelocityToOpticalFlow_Gain/1
  Delay3/1 -> opticalFlow_datout/1

== system sim_quadrotor_2018/ReferenceValueServer/If Action Subsystem ==
  In1 : Inport
  Action Port : ActionPort  ActionType=then
  Out1 : Outport
  wires:
  In1/1 -> Out1/1

== system sim_quadrotor_2018/ReferenceValueServer/If Action Subsystem1 ==
  In1 : Inport
  Action Port : ActionPort  ActionType=then
  Out1 : Outport
  wires:
  In1/1 -> Out1/1

== system sim_quadrotor_2018/ReferenceValueServer/If Action Subsystem2 ==
  In1 : Inport
  Action Port : ActionPort  ActionType=then
  Out1 : Outport
  wires:
  In1/1 -> Out1/1

== system sim_quadrotor_2018/ReferenceValueServer/If Action Subsystem3 ==
  In1 : Inport
  Action Port : ActionPort  ActionType=elseif
  Out1 : Outport
  wires:
  In1/1 -> Out1/1

== system sim_quadrotor_2018/ReferenceValueServer/If Action Subsystem4 ==
  In1 : Inport
  Action Port : ActionPort  ActionType=elseif
  Out1 : Outport
  wires:
  In1/1 -> Out1/1

== system sim_quadrotor_2018/ReferenceValueServer/If Action Subsystem5 ==
  In1 : Inport
  Action Port : ActionPort  ActionType=then
  Out1 : Outport
  wires:
  In1/1 -> Out1/1

== system sim_quadrotor_2018/ReferenceValueServer/If Action Subsystem6 ==
  In1 : Inport
  Action Port : ActionPort  ActionType=then
  Out1 : Outport
  wires:
  In1/1 -> Out1/1

== system sim_quadrotor_2018/ReferenceValueServer/If Action Subsystem7 ==
  In1 : Inport
  Action Port : ActionPort  ActionType=elseif
  Out1 : Outport
  wires:
  In1/1 -> Out1/1

== system sim_quadrotor_2018/Drone_Compensator/ControllerLQR/FullstateController ==
  note: IMPLEMENT FULLSTATE-
      | CONTROLLER HERE
  state_error_datin : Inport
  "A " : Constant  Value=|  VectorParams1D=off
      | [0	0	0	0	0	0	1.00000000000000	0	0	0	0	0
      | 0	0	0	0	0	0	0	1.00000000000000	0	0	0	0
      | 0	0	0	0	0	0	0	0	1.00000000000000	0	0	0
      | 0	0	0	0	0	0	0	0	0	0	0	1.00000000000000
      | 0	0	0	0	0	0	0	0	0	0	1.00000000000000	0
      | 0	0	0	0	0	0	0	0	0	1.00000000000000	0	0
      | 0	0	0	0	-9.80999999983650	0	-0.0644051820480064	0	0	0	0.139009950032610	0
      | 0	0	0	0	0	9.80999999983650	3.94368000217969e-18	-0.0644051820480064	0	-0.139009950032610	-6.26098637146038e-20	-1.52055259660483e-19
      | 0	0	0	0	0	0	0	0	0	0	0	0
      | 0	0	0	0	0	0	0	-1.01355355109772	0	-2.18761944196916	0	0
      | 0	0	0	0	0	0	0.755758408753299	0	0	0	-1.63120319259874	0
      | 0	0	0	0	0	0	0	0	0	1.51387374186132e-16	0	-0.124838403164601]
  B : Constant  Value=|  VectorParams1D=off
      | [0	0	0	0
      | 0	0	0	0
      | 0	0	0	0
      | 0	0	0	0
      | 0	0	0	0
      | 0	0	0	0
      | 0	0	0	0
      | 0	0	0	0
      | -0.00960712392230772	0.00960712392230772	-0.00960712392230772	0.00960712392213385
      | 0.420192001834280	0.420192001834280	-0.420192001834280	-0.420192001834280
      | 0.313317079628604	-0.313317079628604	-0.313317079628604	0.313317079628604
      | -0.0115436310307942	-0.0115436310307942	-0.0115436310307942	-0.0115436310307942]
  Constant : Constant  Value=|  VectorParams1D=off
      | [-8.49718577324068	8.49718577324278	-25.4915573197690	-35.4049407217802	90.0682783196400	89.1568450104141	-11.6214164668536	11.5626871891982	-36.4857972458732	26.1882849112338	26.8528174312964	-44.1008245485000
      | 8.49718577324076	8.49718577324069	25.4915573196879	-35.4049407219011	-90.0682783196407	89.1568450104006	11.6214164668537	11.5626871892001	36.4857972458205	26.1882849112264	-26.8528174312965	-44.1008245487244
      | 8.49718577324275	-8.49718577324067	-25.4915573197688	-35.4049407217802	-90.0682783196551	-89.1568450104008	11.6214164668516	-11.5626871892001	-36.4857972458735	-26.1882849112264	-26.8528174313063	-44.1008245484999
      | -8.49718577324285	-8.49718577324278	25.4915573196756	-35.4049407219011	90.0682783196561	-89.1568450104140	-11.6214164668518	-11.5626871891982	36.4857972458054	-26.1882849112338	26.8528174313064	-44.1008245487245]
  K_lqr_toMotorcmd_slow : Constant  Value=|  VectorParams1D=off
      | [-11.3010583936794	11.3010583936810	-11.3010583936898	-47.0877433069619	118.606403302530	117.689229642168	-15.5706954566703	15.5112876366907	-24.4160285913130	34.5954570321764	35.2626383735406	-53.8321197902419
      | 11.3010583936794	11.3010583936790	11.3010583936727	-47.0877433070400	-118.606403302531	117.689229642160	15.5706954566704	15.5112876366922	24.4160285913003	34.5954570321714	-35.2626383735406	-53.8321197904123
      | 11.3010583936816	-11.3010583936788	-11.3010583936893	-47.0877433069617	-118.606403302539	-117.689229642159	15.5706954566690	-15.5112876366920	-24.4160285913129	-34.5954570321714	-35.2626383735473	-53.8321197902418
      | -11.3010583936815	-11.3010583936811	11.3010583936690	-47.0877433070397	118.606403302539	-117.689229642168	-15.5706954566690	-15.5112876366908	24.4160285912932	-34.5954570321764	35.2626383735473	-53.8321197904121]
  MATLAB Function : MATLAB Function  TreatAsAtomicUnit=on
  motors_refout : Outport
  wires:
  state_error_datin/1 -> MATLAB Function/2(x)
  MATLAB Function/1(u) -> motors_refout/1
  Constant/1 -> MATLAB Function/1(K)

== system sim_quadrotor_2018/Drone_Compensator/ControllerLQR/SysteminputConverter ==
  note: NOTE: The Systeminputconverter takes care of two things:
      | 1) During take off, adjust the total thrust proposed by the controller
      | 2) Translate the "mechanical" system inputs (total thrust, torques around body-frame x-y-z-axes) to actual motor commands.
      | This R4->R4 mapping is a simple bijective function and does not have any dynamics. This allows us to design the controller with more intuitive "mechanical inputs" (total thrust, torques) and later simple map these to actual motor commands.
  takeoffphase_flagin : Inport
  motors_refin : Inport  Port=2
  ControlMixer : Subsystem
  Conversion Motorcommands To TotalThrust and Torques : Subsystem
  Demux3 : Demux
  Takeoffphase_Thrustadjustment : Subsystem
  Thrust2Motorcmd : Subsystem
  motors_refout : Outport
  wires:
  takeoffphase_flagin/1 -> Takeoffphase_Thrustadjustment/1(takeoffphase_flagin)
  Takeoffphase_Thrustadjustment/1(totThrust_refout) -> ControlMixer/1(T_refin)
  Demux3/1 -> Takeoffphase_Thrustadjustment/2(totThrustbyController_refin)
  Demux3/4 -> ControlMixer/4(tau_roll)
  Demux3/3 -> ControlMixer/3(tau_pitch)
  Demux3/2 -> ControlMixer/2(tau_yaw)
  ControlMixer/1(thrusts_refout) -> Thrust2Motorcmd/1(thrusts_refin)
  Thrust2Motorcmd/1(motors_refout) -> motors_refout/1
  motors_refin/1 -> Conversion Motorcommands To TotalThrust and Torques/1(motors_refin)
  Conversion Motorcommands To TotalThrust and Torques/1(u_tthrust_torques) -> Demux3/1

== system sim_quadrotor_2018/Drone_Compensator/ControllerLQR/statesReferences ==
  note: orietation-only control reference
  note: Full-pose-reference
  note: NOTE: When we want the drone to reach and maintain a given non-zero orientation,
      | we obviously do not care about errors in x-y-position . A fullstate-feedback controller, however, acts
      | on the full state-error. To avoid influences of a x-y-position error (because in orientation-only-control we don't care about it),
      | we set the x-y-reference-position to the current postition estimate (so we get a zero "x-y-position" error).
  pos_refin : Inport
  orient_refin : Inport  Port=2
  controlModePosVSOrient_flagin : Inport  Port=3
  states_estimin : Inport  Port=4
  Bus Selector : BusSelector  OutputSignals=X,Y
  Bus Selector1 : BusSelector  OutputSignals=dx,dy
  Mux1 : Mux  Inputs=3
  Mux3 : Mux
  Mux4 : Mux
  Mux5 : Mux  Inputs=3
  PosVSOrient_Switch : Switch  Criteria=u2 > Threshold
  Selector : Selector  InputPortWidth=3  IndexOptions=Index vector (dialog)  Indices=[3]  OutputSizes=1
  dz_ref : Constant  Value=0
  velocitiesPos_ref : Constant  Value=[0;0;0]
  velocitiesRot_ref : Constant  Value=[0;0;0]
  states_refout : Outport
  wires:
  dz_ref/1 -> Mux1/3
  Mux1/1 -> Mux4/3
  Bus Selector1/2 -> Mux1/2  "<dy>"
  Bus Selector1/1 -> Mux1/1  "<dx>"
  Mux5/1 -> Mux4/1
  Mux4/1 -> PosVSOrient_Switch/3
  Bus Selector/2 -> Mux5/2  "<Y>"
  Bus Selector/1 -> Mux5/1  "<X>"
  Mux3/1 -> PosVSOrient_Switch/1
  controlModePosVSOrient_flagin/1 -> PosVSOrient_Switch/2
  Selector/1 -> Mux5/3
  PosVSOrient_Switch/1 -> states_refout/1
  velocitiesRot_ref/1 -> Mux4/4, Mux3/4
  velocitiesPos_ref/1 -> Mux3/3
  states_estimin/1 -> Bus Selector/1, Bus Selector1/1
  orient_refin/1 -> Mux4/2, Mux3/2
  pos_refin/1 -> Mux3/1, Selector/1

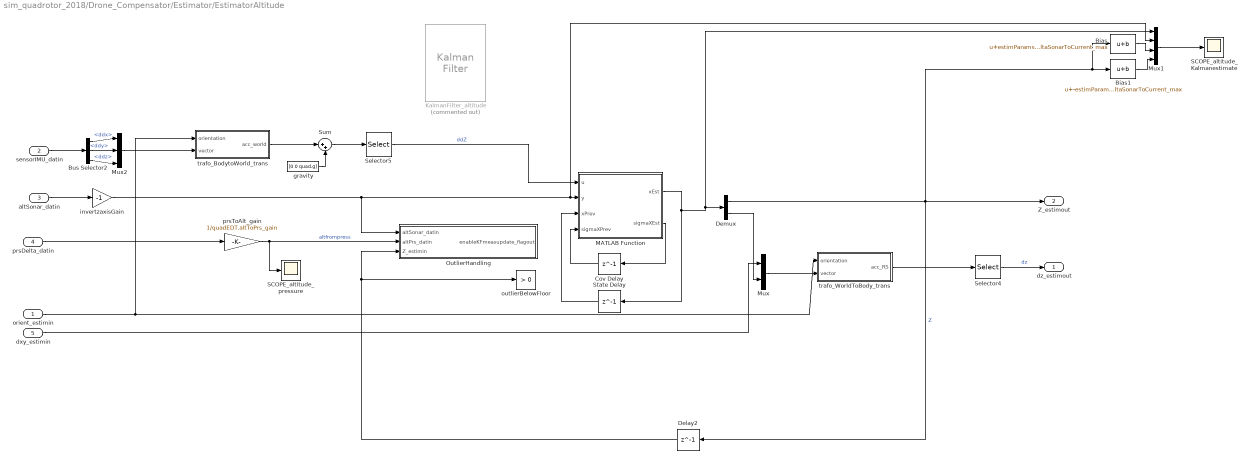
== system sim_quadrotor_2018/Drone_Compensator/Estimator/EstimatorAltitude ==
  orient_estimin : Inport
  sensorIMU_datin : Inport  Port=2
  altSonar_datin : Inport  Port=3
  prsDelta_datin : Inport  Port=4
  dxy_estimin : Inport  Port=5
  Bias : Bias  Bias=estimParams.alt.deltaSonarToCurrent_max
  Bias1 : Bias  Bias=-estimParams.alt.deltaSonarToCurrent_max
  Bus Selector2 : BusSelector  OutputSignals=ddx,ddy,ddz
  Cov Delay : Delay  DelayLength=1  InitialCondition=sigmaX0
  Delay2 : Delay  DelayLength=1  InitialCondition=0
  Demux : Demux  Outputs=2
  KalmanFilter_altitude : ctrlSharedLib/Kalman Filter  Commented=on  TimeDomain=Discrete-Time  UseCurrentEstimator=on  ModelSource=Individual A, B, C, D matrices  ModelSourceVariable=sys  A=[1 quadEDT.sampletime; 0 1]  B=[0;quadEDT.sampletime]  C=[1 0]  D=[0]  NumberOfStates=2  NumberOfInputs=2  NumberOfOutputs=2  InitialEstimateSource=Dialog  X0=[-0.046 0]  P0=10  UseK=off  UseGH=on  NumberOfProcessNoiseInputs=2  G=estimParams.alt.kf.G  TimeInvariantG=on  H=estimParams.alt.kf.H  TimeInvariantH=on  Q=estimParams.alt.kf.Q  TimeInvariantQ=on  R=estimParams.alt.kf.R  TimeInvariantR=on  N=estimParams.alt.kf.N  TimeInvariantN=on  AddInputPort=on  AddEnablePort=on  ExternalReset=Level hold  OutputEstimatedY=off  OutputP=off  Ts=-1
      settings: SourceProductBaseCode=CT
  MATLAB Function : MATLAB Function  TreatAsAtomicUnit=on
  Mux : Mux  Inputs=2
  Mux1 : Mux
  Mux2 : Mux  Inputs=3
  OutlierHandling : Subsystem
  SCOPE_altitude_Kalmanestimate : Scope
  SCOPE_altitude_pressure : Scope
  Selector4 : Selector  InputPortWidth=3  IndexOptions=Index vector (dialog)  Indices=[3]  OutputSizes=1
  Selector5 : Selector  InputPortWidth=3  IndexOptions=Index vector (dialog)  Indices=[3]  OutputSizes=1
  State Delay : Delay  DelayLength=1  InitialCondition=x0
  Sum : Sum  Inputs=|++
  gravity : Constant  Value=[0 0 quad.g]
  invertzaxisGain : Gain  Gain=-1
  outlierBelowFloor : simulink/Logic and Bit Operations/Compare To Constant  relop=>  const=0  OutDataTypeStr=boolean
  prsToAlt_gain : Gain  Gain=1/quadEDT.altToPrs_gain
  trafo_BodytoWorld_trans : MATLAB Function  TreatAsAtomicUnit=on
  trafo_WorldToBody_trans : MATLAB Function  TreatAsAtomicUnit=on
  dz_estimout : Outport
  Z_estimout : Outport  Port=2
  wires:
  orient_estimin/1 -> trafo_BodytoWorld_trans/1(orientation), trafo_WorldToBody_trans/1(orientation)
  altSonar_datin/1 -> invertzaxisGain/1
  trafo_BodytoWorld_trans/1(acc_world) -> Sum/1
  gravity/1 -> Sum/2
  Sum/1 -> Selector5/1
  MATLAB Function/1(xEst) -> Mux1/1, Demux/1, State Delay/1
  Mux/1 -> trafo_WorldToBody_trans/2(vector)
  Selector5/1 -> MATLAB Function/1(u)  "ddZ"
  invertzaxisGain/1 -> Mux1/2, MATLAB Function/2(y), OutlierHandling/1(altSonar_datin)
  Demux/1 -> Bias1/1, Bias/1, Delay2/1, Z_estimout/1  "Z"
  Selector4/1 -> dz_estimout/1  "dz"
  Demux/2 -> Mux/2
  Mux1/1 -> SCOPE_altitude_Kalmanestimate/1
  Bias/1 -> Mux1/3
  Bias1/1 -> Mux1/4
  prsDelta_datin/1 -> prsToAlt_gain/1
  prsToAlt_gain/1 -> SCOPE_altitude_pressure/1, OutlierHandling/2(altPrs_datin)  "altfrompress"
  Delay2/1 -> outlierBelowFloor/1, OutlierHandling/3(Z_estimin)
  dxy_estimin/1 -> Mux/1
  trafo_WorldToBody_trans/1(acc_RS) -> Selector4/1
  Bus Selector2/1 -> Mux2/1  "<ddx>"
  Bus Selector2/2 -> Mux2/2  "<ddy>"
  Bus Selector2/3 -> Mux2/3  "<ddz>"
  sensorIMU_datin/1 -> Bus Selector2/1
  Mux2/1 -> trafo_BodytoWorld_trans/2(vector)
  State Delay/1 -> MATLAB Function/3(xPrev)
  Cov Delay/1 -> MATLAB Function/4(sigmaXPrev)
  MATLAB Function/2(sigmaXEst) -> Cov Delay/1

== system sim_quadrotor_2018/Drone_Compensator/Estimator/EstimatorXYPosition ==
  opticalFlow_datin : Inport
  controlModePosVSOrient_flagin : Inport  Port=2
  usePosVIS_flagin : Inport  Port=3
  posVIS_datin : Inport  Port=4
  sensorIMU_datin : Inport  Port=5
  orient_estimin : Inport  Port=6
  Z_estimin : Inport  Port=7
  dz_estimin : Inport  Port=8
  EstimatorVelocity : Subsystem
  EstimatorXYPosition : Subsystem
  XY_estimout : Outport
  dxy_estimout : Outport  Port=2
  wires:
  orient_estimin/1 -> EstimatorVelocity/4(orient_estimin), EstimatorXYPosition/2(orient_estimin)
  EstimatorVelocity/1(dxy_estimout) -> EstimatorXYPosition/1(dxy_estimin), dxy_estimout/1
  opticalFlow_datin/1 -> EstimatorVelocity/1(opticalFlow_datin)
  sensorIMU_datin/1 -> EstimatorVelocity/3(sensorIMU_datin)
  Z_estimin/1 -> EstimatorVelocity/2(Z_estimin)
  controlModePosVSOrient_flagin/1 -> EstimatorXYPosition/3(controlModePosVSOrient_flagin)
  dz_estimin/1 -> EstimatorXYPosition/4(dz_estimin)
  posVIS_datin/1 -> EstimatorXYPosition/5(posVIS_datin)
  usePosVIS_flagin/1 -> EstimatorXYPosition/6(usePosVIS_flagin)
  EstimatorXYPosition/1(XY_estimout) -> XY_estimout/1

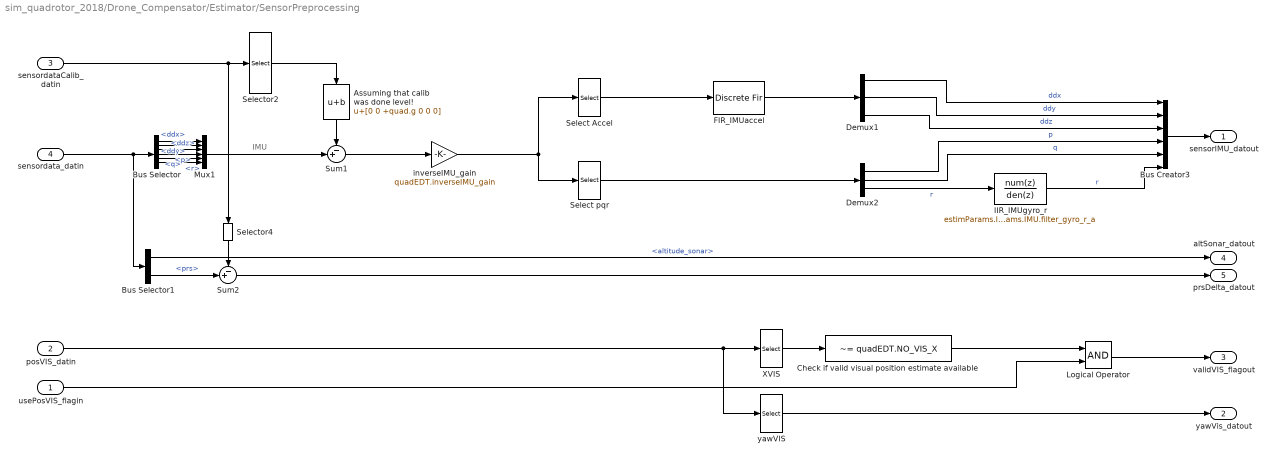
== system sim_quadrotor_2018/Drone_Compensator/Estimator/SensorPreprocessing ==
  note: IMU
  usePosVIS_flagin : Inport
  posVIS_datin : Inport  Port=2
  sensordataCalib_datin : Inport  Port=3
  sensordata_datin : Inport  Port=4
  Assuming that calib was done level! : Bias  Bias=[0 0 +quad.g 0 0 0]
  Bus Creator3 : BusCreator  Inputs=6
  Bus Selector : BusSelector  OutputSignals=ddx,ddy,ddz,p,q,r
  Bus Selector1 : BusSelector  OutputSignals=altitude_sonar,prs
  Check if valid visual position estimate available : simulink/Logic and Bit Operations/Compare To Constant  relop=~=  const=quadEDT.NO_VIS_X  OutDataTypeStr=boolean
  Demux1 : Demux  Outputs=3
  Demux2 : Demux  Outputs=3
  FIR_IMUaccel : DiscreteFir  Coefficients=estimParams.IMU.filter_accel.Coefficients
  IIR_IMUgyro_r : DiscreteFilter  Numerator=estimParams.IMU.filter_gyro_r_b  Denominator=estimParams.IMU.filter_gyro_r_a
  Logical Operator : Logic  AllPortsSameDT=off  OutDataTypeStr=boolean
  Mux1 : Mux  Inputs=6
  Select Accel : Selector  InputPortWidth=6  IndexOptions=Index vector (dialog)  Indices=[1 2 3]  OutputSizes=1
  Select pqr : Selector  InputPortWidth=6  IndexOptions=Index vector (dialog)  Indices=[4 5 6]  OutputSizes=1
  Selector2 : Selector  InputPortWidth=7  IndexOptions=Index vector (dialog)  Indices=[1:6]  OutputSizes=1
  Selector4 : Selector  InputPortWidth=7  IndexOptions=Index vector (dialog)  Indices=[7]  OutputSizes=1
  Sum1 : Sum  Inputs=-+|
  Sum2 : Sum  Inputs=-+|
  XVIS : Selector  InputPortWidth=4  IndexOptions=Index vector (dialog)  Indices=1  OutputSizes=1
  inverseIMU_gain : Gain  Gain=quadEDT.inverseIMU_gain
  yawVIS : Selector  InputPortWidth=4  IndexOptions=Index vector (dialog)  Indices=4  OutputSizes=1
  sensorIMU_datout : Outport
  yawVis_datout : Outport  Port=2
  validVIS_flagout : Outport  Port=3
  altSonar_datout : Outport  Port=4
  prsDelta_datout : Outport  Port=5
  wires:
  posVIS_datin/1 -> yawVIS/1, XVIS/1
  Bus Creator3/1 -> sensorIMU_datout/1
  Demux1/1 -> Bus Creator3/1  "ddx"
  Demux1/2 -> Bus Creator3/2  "ddy"
  Demux1/3 -> Bus Creator3/3  "ddz"
  Sum1/1 -> inverseIMU_gain/1
  Selector2/1 -> Assuming that calib was done level!/1
  Demux2/1 -> Bus Creator3/4  "p"
  Demux2/2 -> Bus Creator3/5  "q"
  inverseIMU_gain/1 -> Select pqr/1, Select Accel/1
  Select Accel/1 -> FIR_IMUaccel/1
  FIR_IMUaccel/1 -> Demux1/1
  Demux2/3 -> IIR_IMUgyro_r/1  "r"
  IIR_IMUgyro_r/1 -> Bus Creator3/6  "r"
  sensordataCalib_datin/1 -> Selector4/1, Selector2/1
  Bus Selector/1 -> Mux1/1  "<ddx>"
  Bus Selector/2 -> Mux1/2  "<ddy>"
  Bus Selector/3 -> Mux1/3  "<ddz>"
  Bus Selector/4 -> Mux1/4  "<p>"
  Bus Selector/5 -> Mux1/5  "<q>"
  Bus Selector/6 -> Mux1/6  "<r>"
  sensordata_datin/1 -> Bus Selector1/1, Bus Selector/1
  Bus Selector1/1 -> altSonar_datout/1  "<altitude_sonar>"
  Selector4/1 -> Sum2/1
  Bus Selector1/2 -> Sum2/2  "<prs>"
  Sum2/1 -> prsDelta_datout/1
  Mux1/1 -> Sum1/2
  XVIS/1 -> Check if valid visual position estimate available/1
  yawVIS/1 -> yawVis_datout/1
  Logical Operator/1 -> validVIS_flagout/1
  Check if valid visual position estimate available/1 -> Logical Operator/1
  usePosVIS_flagin/1 -> Logical Operator/2
  Assuming that calib was done level!/1 -> Sum1/1
  Select pqr/1 -> Demux2/1
